simulink model "PatternWizard"  (R2020a)
settings: Solver=FixedStepDiscrete  StartTime=0.0  StopTime=10.0  FixedStep=1.0  RelTol=1e-3
values from neighbouring files (symbols this model uses):
  thd = 25    [matlab.mat]
libraries: simulink x1
settings Model: Creator=ashok  LastModifiedBy=ashok

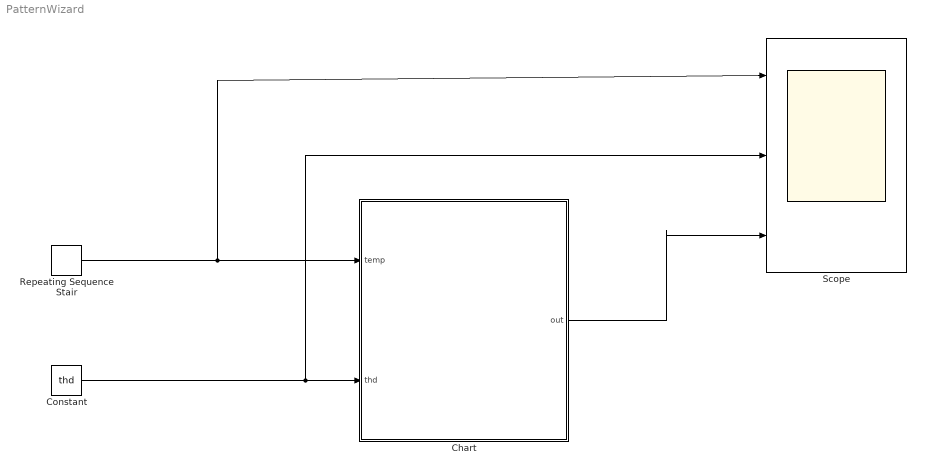
== system PatternWizard ==
  Chart : Stateflow chart  TreatAsAtomicUnit=on
  Constant : Constant  Value=thd
  Repeating Sequence Stair : simulink/Sources/Repeating Sequence Stair  OutValues=temp  tsamp=-1  OutMin=[]  OutMax=[]  OutDataTypeStr=double  OutputDataTypeScalingMode=double  OutDataType=fixdt(0,8)  ConRadixGroup=Best Precision: Vector-wise  OutScaling=2^-12
  Scope : Scope  NumInputPorts=3
  wires:
  Repeating Sequence Stair/1 -> Scope/1, Chart/1(temp)
  Constant/1 -> Scope/2, Chart/2(thd)
  Chart/1(out) -> Scope/3

== stateflow chart PatternWizard/Chart ==
  (default) -> (junction 14) : % Temperature check
  (junction 14) -> (junction 15) [order 1] : [temp > thd]
  (junction 14) -> (junction 16) [order 2]
  (junction 15) -> (junction 20) : {out = -1;}
  (junction 16) -> (junction 17) [order 1] : [temp < thd]
  (junction 16) -> (junction 18) [order 2] : {out = 0;}
  (junction 17) -> (junction 19) : {out = 1;}
  (junction 19) -> (junction 18)
  (junction 20) -> (junction 19)
  (junction 18) -> (junction 21)
  data: temp input; thd input; out output
